simulink model "ss_inter_v3_i"  (R2019a)
settings: Solver=ode14x  StartTime=beginTime  StopTime=.3917  FixedStep=1e-4  RelTol=1e-3  EnableMultiTasking=on
model workspace (MAT data in the model file):
  Ankle_L_D = 1.86999822456
  Ankle_L_S = 0.0237763920936
  Ankle_R_D = 0.0588397140494
  Ankle_R_S = 0.739584271752
  F_C = 0.0618
  F_H = 0.107
  F_I = 0.0129
  F_L = 0.2471
  F_M = 1.2499
  F_W = 0.11
  GRF_HD = 42097.5090581
  GRF_HS = 111995.804745
  GRF_VD = 23523.4518935
  GRF_VS = 88551.3661398
  HAT_I = 4.3688
  HAT_L = 0.549
  HAT_M = 58.9182
  HAT_a = 0.2
  HAT_b = 0.13
  Hip_L_D = 0.00120944164738
  Hip_L_S = 1.91959156409
  Hip_R_D = 0.00174333284727
  Hip_R_S = 0.483982271561
  Knee_L_D = 0.900041230997
  Knee_L_S = 0.0187606009115
  Knee_R_D = 0.0722123401531
  Knee_R_S = 0.341684886913
  M : struct (value not decoded)
  S_I = 0.073
  S_L = 0.447
  S_M = 4.0083
  S_R1 = 0.06
  S_R2 = 0.08
  T_I = 0.2042
  T_L = 0.476
  T_M = 8.62
  T_R1 = 0.08
  T_R2 = 0.1
  beginTime = 0
  bodymass = 86.2
  lagStanceAnkle = [-99.7972 119.6384 39.1959 13.6502 4.806 38.9221]
  lagSwingAnkle = [13.6022 -2.7997 -4.4346 -3.8168 -10.7505 -9.0476]
  lagSwingHip = [-0.8171 -4.531 -6.5727 -10.5819 -21.4348 -39.6754]
  lagSwingKnee = [12.9765 10.8307 12.1552 13.6508 15.8758 16.223]
  p_stance_ankle_i = 1.9958
  p_stance_hip_i = -0.3323
  p_stance_knee_i = -0.8489
  p_swing_ankle_i = -0.4822
  p_swing_hip_i = -0.4475
  p_swing_knee_i = -0.4822
  polyfit_stance_ankle = [14817.0133912 -12307.4669363 2660.6079459 -392.465308084 -22.4679780976]
  polyfit_swing_ankle = [1827062.95885 -2490254.69612 1362128.66207 -378716.545114 54333.2821512 -3279.80936759 -14.4988961426 7.65411149052]
  polyfit_swing_hip = [-165694475.688 242689298.766 -143233708.247 44214448.7429 -7786254.41967 786446.146696 -39221.5649329 184.642317874 42.6030082642]
  polyfit_swing_knee = [-833880.523134 699128.406901 -179568.608041 9158.11345477 2208.69768841 -148.905653355 -15.7767198565]
  w_stance_ankle_i = 1.3
  w_stance_hip_i = 1.44372264721e-05
  w_stance_knee_i = 1.72097647422e-05
  w_swing_ankle_i = -2.2
  w_swing_hip_i = -0.00239916102262
  w_swing_knee_i = -0.00263690015709
  x_planar_p_i = 0
  x_planar_v_i = 0
  y_planar_p_i = 0
  y_planar_v_i = 0
  z_planar_p_i = 0
  z_planar_v_i = 0
values from neighbouring files (symbols this model uses):
  N = 3    [lagdmodel.m]
symbols that are objects in the model workspace (value not decoded): M
undefined symbols (not defined in the file or in its folder): X, Y, Z
libraries: nesl_utility x104, sm_lib x67, fl_lib x24, fl_ps_legacy_lib x14
(part 4 of 4)

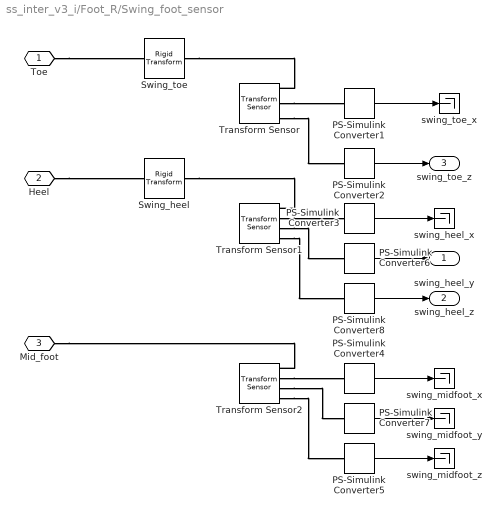
== system ss_inter_v3_i/Foot_R/Swing_foot_sensor ==
  PS-Simulink Converter{1..8} (8 alike) : nesl_utility/PS-Simulink Converter  PhysicalDomain=network_engine_domain  SubClassName=ps_output  LeftPortType=input  RightPortType=output  PseudoPeriodic=off  Frequencies=[]  Unit=1  AffineConversion=off
  Swing_heel : sm_lib/Frames and Transforms/Rigid Transform  TranslationMethod=StandardAxis  TranslationStandardOffset=F_C  TranslationLengthUnit=m  TranslationStandardAxis=-X  TranslationCartesianOffset=[0 0 0]  TranslationROffset=0  TranslationROffsetUnits=m  TranslationZOffset=0  TranslationZOffsetUnits=m  TranslationThetaOffset=0  TranslationThetaOffsetUnits=deg  RotationMethod=None  RotationAngleUnits=deg  RotationStandardAxis=+Z  RotationAngle=0  RotationArbitraryAxis=[0 0 1]  FollAlignAxisA=+X  BaseAlignAxisA=+Y  FollAlignAxisB=+Y  BaseAlignAxisB=+Z  RotationSequenceAxes=FollowerAxes  RotationSequence=XYX  RotationSequenceAngles=[0 0 0]  RotationSequenceAnglesUnits=deg  RotationMatrix=[1 0 0; 0 1 0; 0 0 1]
  Swing_toe : sm_lib/Frames and Transforms/Rigid Transform  TranslationMethod=StandardAxis  TranslationStandardOffset=F_L-F_C  TranslationLengthUnit=m  TranslationStandardAxis=+X  TranslationCartesianOffset=[0 0 0]  TranslationROffset=0  TranslationROffsetUnits=m  TranslationZOffset=0  TranslationZOffsetUnits=m  TranslationThetaOffset=0  TranslationThetaOffsetUnits=deg  RotationMethod=None  RotationAngleUnits=deg  RotationStandardAxis=+Z  RotationAngle=0  RotationArbitraryAxis=[0 0 1]  FollAlignAxisA=+X  BaseAlignAxisA=+Y  FollAlignAxisB=+Y  BaseAlignAxisB=+Z  RotationSequenceAxes=FollowerAxes  RotationSequence=XYX  RotationSequenceAngles=[0 0 0]  RotationSequenceAnglesUnits=deg  RotationMatrix=[1 0 0; 0 1 0; 0 0 1]
  Transform Sensor : sm_lib/Frames and Transforms/Transform Sensor  MeasurementFrame=World  SenseAngle=off  SenseAxis=off  SenseAngle1=off  SenseAngle2=off  SenseAngle3=off  SenseQ=off  SenseR=off  SenseOmegaX=off  SenseOmegaY=off  SenseOmegaZ=off  SenseOmega1=off  SenseOmega2=off  SenseOmega3=off  SenseQDot=off  SenseRDot=off  SenseAlphaX=off  SenseAlphaY=off  SenseAlphaZ=off  SenseAlpha1=off  SenseAlpha2=off  SenseAlpha3=off  SenseQDDot=off  SenseRDDot=off  SenseX=on  SenseY=off  SenseZ=on  SenseRad=off  SenseAzim=off  SenseDist=off  SenseInc=off  SenseXDot=off  SenseYDot=off  SenseZDot=off  SenseRadDot=off  SenseAzimDot=off  SenseDistDot=off  SenseIncDot=off  SenseXDDot=off  SenseYDDot=off  SenseZDDot=off  SenseRadDDot=off  SenseAzimDDot=off  SenseDistDDot=off  SenseIncDDot=off
  Transform Sensor1 : sm_lib/Frames and Transforms/Transform Sensor  MeasurementFrame=World  SenseAngle=off  SenseAxis=off  SenseAngle1=off  SenseAngle2=off  SenseAngle3=off  SenseQ=off  SenseR=off  SenseOmegaX=off  SenseOmegaY=off  SenseOmegaZ=off  SenseOmega1=off  SenseOmega2=off  SenseOmega3=off  SenseQDot=off  SenseRDot=off  SenseAlphaX=off  SenseAlphaY=off  SenseAlphaZ=off  SenseAlpha1=off  SenseAlpha2=off  SenseAlpha3=off  SenseQDDot=off  SenseRDDot=off  SenseX=on  SenseY=on  SenseZ=on  SenseRad=off  SenseAzim=off  SenseDist=off  SenseInc=off  SenseXDot=off  SenseYDot=off  SenseZDot=off  SenseRadDot=off  SenseAzimDot=off  SenseDistDot=off  SenseIncDot=off  SenseXDDot=off  SenseYDDot=off  SenseZDDot=off  SenseRadDDot=off  SenseAzimDDot=off  SenseDistDDot=off  SenseIncDDot=off
  Transform Sensor2 : sm_lib/Frames and Transforms/Transform Sensor  MeasurementFrame=World  SenseAngle=off  SenseAxis=off  SenseAngle1=off  SenseAngle2=off  SenseAngle3=off  SenseQ=off  SenseR=off  SenseOmegaX=off  SenseOmegaY=off  SenseOmegaZ=off  SenseOmega1=off  SenseOmega2=off  SenseOmega3=off  SenseQDot=off  SenseRDot=off  SenseAlphaX=off  SenseAlphaY=off  SenseAlphaZ=off  SenseAlpha1=off  SenseAlpha2=off  SenseAlpha3=off  SenseQDDot=off  SenseRDDot=off  SenseX=on  SenseY=on  SenseZ=on  SenseRad=off  SenseAzim=off  SenseDist=off  SenseInc=off  SenseXDot=off  SenseYDot=off  SenseZDot=off  SenseRadDot=off  SenseAzimDot=off  SenseDistDot=off  SenseIncDot=off  SenseXDDot=off  SenseYDDot=off  SenseZDDot=off  SenseRadDDot=off  SenseAzimDDot=off  SenseDistDDot=off  SenseIncDDot=off
  swing_heel_x : Terminator
  swing_midfoot_x : Terminator
  swing_midfoot_y : Terminator
  swing_midfoot_z : Terminator
  swing_toe_x : Terminator
  Toe : PMIOPort  Side=Left
  Heel : PMIOPort  Port=2  Side=Left
  Mid_foot : PMIOPort  Port=3  Side=Left
  swing_heel_y : Outport
  swing_heel_z : Outport  Port=2
  swing_toe_z : Outport  Port=3
  wires:
  PS-Simulink Converter1/1 -> swing_toe_x/1
  PS-Simulink Converter2/1 -> swing_toe_z/1
  PS-Simulink Converter3/1 -> swing_heel_x/1
  PS-Simulink Converter6/1 -> swing_heel_y/1
  PS-Simulink Converter4/1 -> swing_midfoot_x/1
  PS-Simulink Converter7/1 -> swing_midfoot_y/1
  PS-Simulink Converter5/1 -> swing_midfoot_z/1
  PS-Simulink Converter8/1 -> swing_heel_z/1
  connections:
  Swing_heel/RConn1 -- Transform Sensor1/RConn1
  Swing_toe/RConn1 -- Transform Sensor/RConn1
  Heel/RConn1 -- Swing_heel/LConn1
  Toe/RConn1 -- Swing_toe/LConn1
  Mid_foot/RConn1 -- Transform Sensor2/RConn1
  Transform Sensor2/RConn2 -- PS-Simulink Converter4/LConn1
  Transform Sensor/RConn2 -- PS-Simulink Converter1/LConn1
  Transform Sensor/RConn3 -- PS-Simulink Converter2/LConn1
  Transform Sensor1/RConn2 -- PS-Simulink Converter3/LConn1
  Transform Sensor1/RConn3 -- PS-Simulink Converter6/LConn1
  Transform Sensor2/RConn4 -- PS-Simulink Converter5/LConn1
  Transform Sensor2/RConn3 -- PS-Simulink Converter7/LConn1
  Transform Sensor1/RConn4 -- PS-Simulink Converter8/LConn1

== system ss_inter_v3_i/HAT/COMCal ==
  COM Energy Calc : Subsystem
  PS-S : nesl_utility/PS-Simulink Converter  PhysicalDomain=network_engine_domain  SubClassName=ps_output  LeftPortType=input  RightPortType=output  PseudoPeriodic=off  Frequencies=[]  Unit=1  AffineConversion=off
  Transform Sensor : sm_lib/Frames and Transforms/Transform Sensor  MeasurementFrame=World  SenseAngle=off  SenseAxis=off  SenseAngle1=off  SenseAngle2=off  SenseAngle3=off  SenseQ=off  SenseR=off  SenseOmegaX=off  SenseOmegaY=off  SenseOmegaZ=off  SenseOmega1=off  SenseOmega2=off  SenseOmega3=off  SenseQDot=off  SenseRDot=off  SenseAlphaX=off  SenseAlphaY=off  SenseAlphaZ=off  SenseAlpha1=off  SenseAlpha2=off  SenseAlpha3=off  SenseQDDot=off  SenseRDDot=off  SenseX=off  SenseY=off  SenseZ=on  SenseRad=off  SenseAzim=off  SenseDist=off  SenseInc=off  SenseXDot=on  SenseYDot=on  SenseZDot=on  SenseRadDot=off  SenseAzimDot=off  SenseDistDot=off  SenseIncDot=off  SenseXDDot=off  SenseYDDot=off  SenseZDDot=off  SenseRadDDot=off  SenseAzimDDot=off  SenseDistDDot=off  SenseIncDDot=off
  Conn2 : PMIOPort  Side=Left
  vCOM : Outport
  COM Energy : Outport  Port=2
  wires:
  COM Energy Calc/1(Out1) -> COM Energy/1
  PS-S/1 -> vCOM/1
  connections:
  COM Energy Calc/LConn4 -- Transform Sensor/RConn5
  COM Energy Calc/LConn2 -- Transform Sensor/RConn3
  COM Energy Calc/LConn1 -- Transform Sensor/RConn2
  Transform Sensor/RConn4 -- COM Energy Calc/LConn3 -- PS-S/LConn1
  Transform Sensor/RConn1 -- Conn2/RConn1

== system ss_inter_v3_i/Hip_L_Actuation/Hard_Stop_Hip_L ==
  Mechanical Rotational Reference : fl_lib/Mechanical/Rotational Elements/Mechanical Rotational Reference
  Rotational Simscape Intf (Library Block) : Subsystem
  Rotational Hard Stop : fl_lib/Mechanical/Rotational Elements/Rotational Hard Stop  upper_bnd=upper_bound rad  lower_bnd=lower_bound rad  stiff_up=contact_stiffness N*m/rad  stiff_low=contact_stiffness N*m/rad  D_up=contact_damping N*m/(rad/s)  D_low=contact_damping N*m/(rad/s)  model=3  transition=0.001 rad  w_specify=off  w_priority=None  w=0 rad/s  w_nominal_specify=off  w_nominal_unit=rad/s  w_nominal_value=1  t_specify=off  t_priority=None  t=0 N*m  t_nominal_specify=off  t_nominal_unit=N*m  t_nominal_value=1  phi_specify=on  phi_priority=High  phi=initial_angular_position rad  phi_nominal_specify=off  phi_nominal_unit=rad  phi_nominal_value=1
      settings: SourceProductName=Simscape  SourceProductBaseCode=SS
  T : PMIOPort  Side=Right
  w : PMIOPort  Port=2  Side=Left
  connections:
  Rotational Simscape Intf (Library Block)/LConn2 -- Rotational Hard Stop/LConn1 -- Mechanical Rotational Reference/LConn1
  Rotational Hard Stop/RConn1 -- Rotational Simscape Intf (Library Block)/RConn2
  w/RConn1 -- Rotational Simscape Intf (Library Block)/LConn1
  Rotational Simscape Intf (Library Block)/RConn1 -- T/RConn1

== system ss_inter_v3_i/Hip_R_Actuation/Hard_Stop_Hip_R ==
  Mechanical Rotational Reference : fl_lib/Mechanical/Rotational Elements/Mechanical Rotational Reference
  Rotational Simscape Intf (Library Block) : Subsystem
  Rotational Hard Stop : fl_lib/Mechanical/Rotational Elements/Rotational Hard Stop  upper_bnd=upper_bound rad  lower_bnd=lower_bound rad  stiff_up=contact_stiffness N*m/rad  stiff_low=contact_stiffness N*m/rad  D_up=contact_damping N*m/(rad/s)  D_low=contact_damping N*m/(rad/s)  model=3  transition=0.001 rad  w_specify=off  w_priority=None  w=0 rad/s  w_nominal_specify=off  w_nominal_unit=rad/s  w_nominal_value=1  t_specify=off  t_priority=None  t=0 N*m  t_nominal_specify=off  t_nominal_unit=N*m  t_nominal_value=1  phi_specify=on  phi_priority=High  phi=initial_angular_position rad  phi_nominal_specify=off  phi_nominal_unit=rad  phi_nominal_value=1
      settings: SourceProductName=Simscape  SourceProductBaseCode=SS
  T : PMIOPort  Side=Right
  w : PMIOPort  Port=2  Side=Left
  connections:
  Rotational Simscape Intf (Library Block)/LConn2 -- Rotational Hard Stop/LConn1 -- Mechanical Rotational Reference/LConn1
  Rotational Hard Stop/RConn1 -- Rotational Simscape Intf (Library Block)/RConn2
  w/RConn1 -- Rotational Simscape Intf (Library Block)/LConn1
  Rotational Simscape Intf (Library Block)/RConn1 -- T/RConn1

== system ss_inter_v3_i/Knee_L_Actuation/Hard_Stop_Knee_L ==
  Mechanical Rotational Reference : fl_lib/Mechanical/Rotational Elements/Mechanical Rotational Reference
  Rotational Simscape Intf (Library Block) : Subsystem
  Rotational Hard Stop : fl_lib/Mechanical/Rotational Elements/Rotational Hard Stop  upper_bnd=upper_bound rad  lower_bnd=lower_bound rad  stiff_up=contact_stiffness N*m/rad  stiff_low=contact_stiffness N*m/rad  D_up=contact_damping N*m/(rad/s)  D_low=contact_damping N*m/(rad/s)  model=3  transition=0.001 rad  w_specify=off  w_priority=None  w=0 rad/s  w_nominal_specify=off  w_nominal_unit=rad/s  w_nominal_value=1  t_specify=off  t_priority=None  t=0 N*m  t_nominal_specify=off  t_nominal_unit=N*m  t_nominal_value=1  phi_specify=on  phi_priority=High  phi=initial_angular_position rad  phi_nominal_specify=off  phi_nominal_unit=rad  phi_nominal_value=1
      settings: SourceProductName=Simscape  SourceProductBaseCode=SS
  T : PMIOPort  Side=Right
  w : PMIOPort  Port=2  Side=Left
  connections:
  Rotational Simscape Intf (Library Block)/RConn1 -- T/RConn1
  w/RConn1 -- Rotational Simscape Intf (Library Block)/LConn1
  Rotational Hard Stop/RConn1 -- Rotational Simscape Intf (Library Block)/RConn2
  Mechanical Rotational Reference/LConn1 -- Rotational Hard Stop/LConn1 -- Rotational Simscape Intf (Library Block)/LConn2

== system ss_inter_v3_i/Knee_R_Actuation/Hard_Stop_Knee_L1 ==
  Mechanical Rotational Reference : fl_lib/Mechanical/Rotational Elements/Mechanical Rotational Reference
  Rotational Simscape Intf (Library Block) : Subsystem
  Rotational Hard Stop : fl_lib/Mechanical/Rotational Elements/Rotational Hard Stop  upper_bnd=upper_bound rad  lower_bnd=lower_bound rad  stiff_up=contact_stiffness N*m/rad  stiff_low=contact_stiffness N*m/rad  D_up=contact_damping N*m/(rad/s)  D_low=contact_damping N*m/(rad/s)  model=3  transition=0.001 rad  w_specify=off  w_priority=None  w=0 rad/s  w_nominal_specify=off  w_nominal_unit=rad/s  w_nominal_value=1  t_specify=off  t_priority=None  t=0 N*m  t_nominal_specify=off  t_nominal_unit=N*m  t_nominal_value=1  phi_specify=on  phi_priority=High  phi=initial_angular_position rad  phi_nominal_specify=off  phi_nominal_unit=rad  phi_nominal_value=1
      settings: SourceProductName=Simscape  SourceProductBaseCode=SS
  T : PMIOPort  Side=Right
  w : PMIOPort  Port=2  Side=Left
  connections:
  Rotational Simscape Intf (Library Block)/RConn1 -- T/RConn1
  w/RConn1 -- Rotational Simscape Intf (Library Block)/LConn1
  Rotational Hard Stop/RConn1 -- Rotational Simscape Intf (Library Block)/RConn2
  Mechanical Rotational Reference/LConn1 -- Rotational Hard Stop/LConn1 -- Rotational Simscape Intf (Library Block)/LConn2

== system ss_inter_v3_i/Shank_L/COM Energy Calc1 ==
  Add : Sum  Inputs=3
  Add1 : Sum  Inputs=2
  Constant : Constant  Value=0.5*(S_M)
  Math Function : Math  Operator=square  SaturateOnIntegerOverflow=on
  Math Function1 : Math  Operator=square  SaturateOnIntegerOverflow=on
  Math Function2 : Math  Operator=square  SaturateOnIntegerOverflow=on
  PS-S{1..4} (4 alike) : nesl_utility/PS-Simulink Converter  PhysicalDomain=network_engine_domain  SubClassName=ps_output  LeftPortType=input  RightPortType=output  PseudoPeriodic=off  Frequencies=[]  Unit=1  AffineConversion=off
  Product : Product  Inputs=3
  Product1 : Product
  g : Constant  Value=9.81
  m : Constant  Value=S_M
  h : PMIOPort  Side=Left
  wx : PMIOPort  Port=2  Side=Left
  vy : PMIOPort  Port=3  Side=Left
  vz : PMIOPort  Port=4  Side=Left
  Out1 : Outport
  wires:
  g/1 -> Product/1
  PS-S2/1 -> Math Function1/1
  PS-S3/1 -> Math Function/1
  PS-S4/1 -> Math Function2/1
  Constant/1 -> Product1/2
  Math Function1/1 -> Add/3
  Add1/1 -> Out1/1
  Product1/1 -> Add1/2
  Math Function2/1 -> Add/1
  Add/1 -> Product1/1
  Math Function/1 -> Add/2
  m/1 -> Product/2
  PS-S1/1 -> Product/3
  Product/1 -> Add1/1
  connections:
  PS-S2/LConn1 -- vz/RConn1
  PS-S3/LConn1 -- vy/RConn1
  PS-S1/LConn1 -- h/RConn1
  PS-S4/LConn1 -- wx/RConn1

== system ss_inter_v3_i/Shank_R/COM Energy Calc1 ==
  Add : Sum  Inputs=3
  Add1 : Sum  Inputs=2
  Constant : Constant  Value=0.5*(S_M)
  Math Function : Math  Operator=square  SaturateOnIntegerOverflow=on
  Math Function1 : Math  Operator=square  SaturateOnIntegerOverflow=on
  Math Function2 : Math  Operator=square  SaturateOnIntegerOverflow=on
  PS-S{1..4} (4 alike) : nesl_utility/PS-Simulink Converter  PhysicalDomain=network_engine_domain  SubClassName=ps_output  LeftPortType=input  RightPortType=output  PseudoPeriodic=off  Frequencies=[]  Unit=1  AffineConversion=off
  Product : Product  Inputs=3
  Product1 : Product
  g : Constant  Value=9.81
  m : Constant  Value=S_M
  h : PMIOPort  Side=Left
  wx : PMIOPort  Port=2  Side=Left
  vy : PMIOPort  Port=3  Side=Left
  vz : PMIOPort  Port=4  Side=Left
  Out1 : Outport
  wires:
  g/1 -> Product/1
  PS-S2/1 -> Math Function1/1
  PS-S3/1 -> Math Function/1
  PS-S4/1 -> Math Function2/1
  Constant/1 -> Product1/2
  Math Function1/1 -> Add/3
  Add1/1 -> Out1/1
  Product1/1 -> Add1/2
  Math Function2/1 -> Add/1
  Add/1 -> Product1/1
  Math Function/1 -> Add/2
  m/1 -> Product/2
  PS-S1/1 -> Product/3
  Product/1 -> Add1/1
  connections:
  PS-S2/LConn1 -- vz/RConn1
  PS-S3/LConn1 -- vy/RConn1
  PS-S1/LConn1 -- h/RConn1
  PS-S4/LConn1 -- wx/RConn1

== system ss_inter_v3_i/Thigh_L/COM Energy Calc1 ==
  Add : Sum  Inputs=3
  Add1 : Sum  Inputs=2
  Constant : Constant  Value=0.5*(T_M)
  Math Function : Math  Operator=square  SaturateOnIntegerOverflow=on
  Math Function1 : Math  Operator=square  SaturateOnIntegerOverflow=on
  Math Function2 : Math  Operator=square  SaturateOnIntegerOverflow=on
  PS-S{1..4} (4 alike) : nesl_utility/PS-Simulink Converter  PhysicalDomain=network_engine_domain  SubClassName=ps_output  LeftPortType=input  RightPortType=output  PseudoPeriodic=off  Frequencies=[]  Unit=1  AffineConversion=off
  Product : Product  Inputs=3
  Product1 : Product
  g : Constant  Value=9.81
  m : Constant  Value=T_M
  h : PMIOPort  Side=Left
  wx : PMIOPort  Port=2  Side=Left
  vy : PMIOPort  Port=3  Side=Left
  vz : PMIOPort  Port=4  Side=Left
  Out1 : Outport
  wires:
  g/1 -> Product/1
  PS-S2/1 -> Math Function1/1
  PS-S3/1 -> Math Function/1
  PS-S4/1 -> Math Function2/1
  Constant/1 -> Product1/2
  Math Function1/1 -> Add/3
  Add1/1 -> Out1/1
  Product1/1 -> Add1/2
  Math Function2/1 -> Add/1
  Add/1 -> Product1/1
  Math Function/1 -> Add/2
  m/1 -> Product/2
  PS-S1/1 -> Product/3
  Product/1 -> Add1/1
  connections:
  PS-S2/LConn1 -- vz/RConn1
  PS-S3/LConn1 -- vy/RConn1
  PS-S1/LConn1 -- h/RConn1
  PS-S4/LConn1 -- wx/RConn1

== system ss_inter_v3_i/Thigh_R/COM Energy Calc1 ==
  Add : Sum  Inputs=3
  Add1 : Sum  Inputs=2
  Constant : Constant  Value=0.5*(T_M)
  Math Function : Math  Operator=square  SaturateOnIntegerOverflow=on
  Math Function1 : Math  Operator=square  SaturateOnIntegerOverflow=on
  Math Function2 : Math  Operator=square  SaturateOnIntegerOverflow=on
  PS-S{1..4} (4 alike) : nesl_utility/PS-Simulink Converter  PhysicalDomain=network_engine_domain  SubClassName=ps_output  LeftPortType=input  RightPortType=output  PseudoPeriodic=off  Frequencies=[]  Unit=1  AffineConversion=off
  Product : Product  Inputs=3
  Product1 : Product
  g : Constant  Value=9.81
  m : Constant  Value=T_M
  h : PMIOPort  Side=Left
  wx : PMIOPort  Port=2  Side=Left
  vy : PMIOPort  Port=3  Side=Left
  vz : PMIOPort  Port=4  Side=Left
  Out1 : Outport
  wires:
  g/1 -> Product/1
  PS-S2/1 -> Math Function1/1
  PS-S3/1 -> Math Function/1
  PS-S4/1 -> Math Function2/1
  Constant/1 -> Product1/2
  Math Function1/1 -> Add/3
  Add1/1 -> Out1/1
  Product1/1 -> Add1/2
  Math Function2/1 -> Add/1
  Add/1 -> Product1/1
  Math Function/1 -> Add/2
  m/1 -> Product/2
  PS-S1/1 -> Product/3
  Product/1 -> Add1/1
  connections:
  PS-S2/LConn1 -- vz/RConn1
  PS-S3/LConn1 -- vy/RConn1
  PS-S1/LConn1 -- h/RConn1
  PS-S4/LConn1 -- wx/RConn1

== system ss_inter_v3_i/Ankle_L_Actuation/Hard_Stop_Ankle_L/Rotational Simscape Intf (Library Block) ==
  Ideal Angular Velocity Source : fl_lib/Mechanical/Mechanical Sources/Ideal Angular Velocity Source
  Ideal Torque Sensor : fl_lib/Mechanical/Mechanical Sensors/Ideal Torque Sensor
  w : PMIOPort  Side=Left
  T : PMIOPort  Port=2  Side=Right
  R : PMIOPort  Port=3  Side=Left
  C : PMIOPort  Port=4  Side=Right
  connections:
  w/RConn1 -- Ideal Angular Velocity Source/RConn1
  T/RConn1 -- Ideal Torque Sensor/RConn2
  Ideal Torque Sensor/LConn1 -- Ideal Angular Velocity Source/RConn2
  R/RConn1 -- Ideal Angular Velocity Source/LConn1
  Ideal Torque Sensor/RConn1 -- C/RConn1

== system ss_inter_v3_i/Ankle_R_Actuation/Hard_Stop_Ankle_L1/Rotational Simscape Intf (Library Block) ==
  Ideal Angular Velocity Source : fl_lib/Mechanical/Mechanical Sources/Ideal Angular Velocity Source
  Ideal Torque Sensor : fl_lib/Mechanical/Mechanical Sensors/Ideal Torque Sensor
  w : PMIOPort  Side=Left
  T : PMIOPort  Port=2  Side=Right
  R : PMIOPort  Port=3  Side=Left
  C : PMIOPort  Port=4  Side=Right
  connections:
  w/RConn1 -- Ideal Angular Velocity Source/RConn1
  T/RConn1 -- Ideal Torque Sensor/RConn2
  Ideal Torque Sensor/LConn1 -- Ideal Angular Velocity Source/RConn2
  R/RConn1 -- Ideal Angular Velocity Source/LConn1
  Ideal Torque Sensor/RConn1 -- C/RConn1

== system ss_inter_v3_i/Foot_L/Heel_GRF/Subsystem ==
  Constant : Constant  Value=0
  Constant1 : Constant  Value=0
  Damping : Switch
  Gain : Gain  Gain=-GRF_VS
  Gain1 : Gain  Gain=-GRF_VD
  PS-Simulink Converter : nesl_utility/PS-Simulink Converter  PhysicalDomain=network_engine_domain  SubClassName=ps_output  LeftPortType=input  RightPortType=output  PseudoPeriodic=off  Frequencies=[]  Unit=1  AffineConversion=off
  PS-Simulink Converter1 : nesl_utility/PS-Simulink Converter  PhysicalDomain=network_engine_domain  SubClassName=ps_output  LeftPortType=input  RightPortType=output  PseudoPeriodic=off  Frequencies=[]  Unit=1  AffineConversion=off
  Scope : Scope
  Scope1 : Scope
  Scope2 : Scope
  Simulink-PS Converter : nesl_utility/Simulink-PS Converter  PhysicalDomain=network_engine_domain  SubClassName=ps_input  LeftPortType=input  RightPortType=output  PseudoPeriodic=off  Frequencies=[]  NoiseDistribution=none  NoiseParameters=[]  Unit=1  AffineConversion=off  FilteringAndDerivatives=zero  SimscapeFilterOrder=1  InputFilterTimeConstant=.001  UdotUserProvided=[]
  Spring : Switch
  Sum : Sum  Inputs=|++
  Vertical Force : PMIOPort  Side=Right
  Vertical Position : PMIOPort  Port=2  Side=Left
  Vertical Velocity : PMIOPort  Port=3  Side=Left
  wires:
  Damping/1 -> Sum/2
  Spring/1 -> Sum/1
  PS-Simulink Converter1/1 -> Scope1/1, Gain1/1
  Gain1/1 -> Damping/3
  Constant1/1 -> Damping/1
  Constant/1 -> Spring/1
  Gain/1 -> Spring/3
  PS-Simulink Converter/1 -> Scope/1, Gain/1, Damping/2, Spring/2
  Sum/1 -> Scope2/1, Simulink-PS Converter/1
  connections:
  Vertical Position/RConn1 -- PS-Simulink Converter/LConn1
  Vertical Velocity/RConn1 -- PS-Simulink Converter1/LConn1
  Simulink-PS Converter/RConn1 -- Vertical Force/RConn1

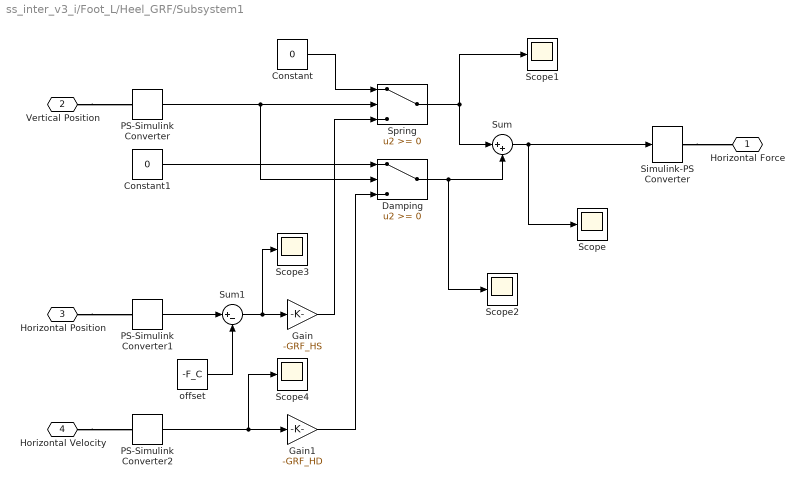
== system ss_inter_v3_i/Foot_L/Heel_GRF/Subsystem1 ==
  Constant : Constant  Value=0
  Constant1 : Constant  Value=0
  Damping : Switch
  Gain : Gain  Gain=-GRF_HS
  Gain1 : Gain  Gain=-GRF_HD
  PS-Simulink Converter : nesl_utility/PS-Simulink Converter  PhysicalDomain=network_engine_domain  SubClassName=ps_output  LeftPortType=input  RightPortType=output  PseudoPeriodic=off  Frequencies=[]  Unit=1  AffineConversion=off
  PS-Simulink Converter1 : nesl_utility/PS-Simulink Converter  PhysicalDomain=network_engine_domain  SubClassName=ps_output  LeftPortType=input  RightPortType=output  PseudoPeriodic=off  Frequencies=[]  Unit=1  AffineConversion=off
  PS-Simulink Converter2 : nesl_utility/PS-Simulink Converter  PhysicalDomain=network_engine_domain  SubClassName=ps_output  LeftPortType=input  RightPortType=output  PseudoPeriodic=off  Frequencies=[]  Unit=1  AffineConversion=off
  Scope{,1..4} (5 alike) : Scope
  Simulink-PS Converter : nesl_utility/Simulink-PS Converter  PhysicalDomain=network_engine_domain  SubClassName=ps_input  LeftPortType=input  RightPortType=output  PseudoPeriodic=off  Frequencies=[]  NoiseDistribution=none  NoiseParameters=[]  Unit=1  AffineConversion=off  FilteringAndDerivatives=zero  SimscapeFilterOrder=1  InputFilterTimeConstant=.001  UdotUserProvided=[]
  Spring : Switch
  Sum : Sum  Inputs=|++
  Sum1 : Sum  Inputs=|+-
  "offset " : Constant  Value=-F_C
  Horizontal Force : PMIOPort  Side=Right
  Vertical Position : PMIOPort  Port=2  Side=Left
  Horizontal Position : PMIOPort  Port=3  Side=Left
  Horizontal Velocity : PMIOPort  Port=4  Side=Left
  wires:
  PS-Simulink Converter/1 -> Spring/2, Damping/2
  Constant/1 -> Spring/1
  Spring/1 -> Scope1/1, Sum/1
  Damping/1 -> Scope2/1, Sum/2
  Constant1/1 -> Damping/1
  PS-Simulink Converter2/1 -> Scope4/1, Gain1/1
  Gain/1 -> Spring/3
  Gain1/1 -> Damping/3
  PS-Simulink Converter1/1 -> Sum1/1
  "offset "/1 -> Sum1/2
  Sum1/1 -> Scope3/1, Gain/1
  Sum/1 -> Simulink-PS Converter/1, Scope/1
  connections:
  Vertical Position/RConn1 -- PS-Simulink Converter/LConn1
  Horizontal Position/RConn1 -- PS-Simulink Converter1/LConn1
  Horizontal Velocity/RConn1 -- PS-Simulink Converter2/LConn1
  Simulink-PS Converter/RConn1 -- Horizontal Force/RConn1

== system ss_inter_v3_i/Foot_L/Toe_GRF/Subsystem ==
  Constant : Constant  Value=0
  Constant1 : Constant  Value=0
  Damping : Switch
  Gain : Gain  Gain=-GRF_VS
  Gain1 : Gain  Gain=-GRF_VD
  PS-Simulink Converter : nesl_utility/PS-Simulink Converter  PhysicalDomain=network_engine_domain  SubClassName=ps_output  LeftPortType=input  RightPortType=output  PseudoPeriodic=off  Frequencies=[]  Unit=1  AffineConversion=off
  PS-Simulink Converter1 : nesl_utility/PS-Simulink Converter  PhysicalDomain=network_engine_domain  SubClassName=ps_output  LeftPortType=input  RightPortType=output  PseudoPeriodic=off  Frequencies=[]  Unit=1  AffineConversion=off
  Scope : Scope
  Scope1 : Scope
  Scope2 : Scope
  Simulink-PS Converter : nesl_utility/Simulink-PS Converter  PhysicalDomain=network_engine_domain  SubClassName=ps_input  LeftPortType=input  RightPortType=output  PseudoPeriodic=off  Frequencies=[]  NoiseDistribution=none  NoiseParameters=[]  Unit=1  AffineConversion=off  FilteringAndDerivatives=zero  SimscapeFilterOrder=1  InputFilterTimeConstant=.001  UdotUserProvided=[]
  Spring : Switch
  Sum : Sum  Inputs=|++
  Vertical Force : PMIOPort  Side=Right
  Vertical Position : PMIOPort  Port=2  Side=Left
  Vertical Velocity : PMIOPort  Port=3  Side=Left
  wires:
  Damping/1 -> Sum/2
  Spring/1 -> Sum/1
  Sum/1 -> Scope2/1, Simulink-PS Converter/1
  PS-Simulink Converter1/1 -> Scope1/1, Gain1/1
  Gain1/1 -> Damping/3
  Constant1/1 -> Damping/1
  Constant/1 -> Spring/1
  Gain/1 -> Spring/3
  PS-Simulink Converter/1 -> Scope/1, Gain/1, Damping/2, Spring/2
  connections:
  Vertical Position/RConn1 -- PS-Simulink Converter/LConn1
  Vertical Velocity/RConn1 -- PS-Simulink Converter1/LConn1
  Simulink-PS Converter/RConn1 -- Vertical Force/RConn1

== system ss_inter_v3_i/Foot_L/Toe_GRF/Subsystem1 ==
  Constant : Constant  Value=0
  Constant1 : Constant  Value=0
  Damping : Switch
  Gain : Gain  Gain=-GRF_HS
  Gain1 : Gain  Gain=-GRF_HD
  PS-Simulink Converter : nesl_utility/PS-Simulink Converter  PhysicalDomain=network_engine_domain  SubClassName=ps_output  LeftPortType=input  RightPortType=output  PseudoPeriodic=off  Frequencies=[]  Unit=1  AffineConversion=off
  PS-Simulink Converter1 : nesl_utility/PS-Simulink Converter  PhysicalDomain=network_engine_domain  SubClassName=ps_output  LeftPortType=input  RightPortType=output  PseudoPeriodic=off  Frequencies=[]  Unit=1  AffineConversion=off
  PS-Simulink Converter2 : nesl_utility/PS-Simulink Converter  PhysicalDomain=network_engine_domain  SubClassName=ps_output  LeftPortType=input  RightPortType=output  PseudoPeriodic=off  Frequencies=[]  Unit=1  AffineConversion=off
  Scope : Scope
  Simulink-PS Converter : nesl_utility/Simulink-PS Converter  PhysicalDomain=network_engine_domain  SubClassName=ps_input  LeftPortType=input  RightPortType=output  PseudoPeriodic=off  Frequencies=[]  NoiseDistribution=none  NoiseParameters=[]  Unit=1  AffineConversion=off  FilteringAndDerivatives=zero  SimscapeFilterOrder=1  InputFilterTimeConstant=.001  UdotUserProvided=[]
  Spring : Switch
  Sum : Sum  Inputs=|++
  Sum1 : Sum  Inputs=|+-
  "offset " : Constant  Value=F_L-F_C
  Horizontal Force : PMIOPort  Side=Right
  Vertical Position : PMIOPort  Port=2  Side=Left
  Horizontal Position : PMIOPort  Port=3  Side=Left
  Horizontal Velocity : PMIOPort  Port=4  Side=Left
  wires:
  PS-Simulink Converter/1 -> Spring/2, Damping/2
  Constant/1 -> Spring/1
  Sum/1 -> Scope/1, Simulink-PS Converter/1
  Spring/1 -> Sum/1
  Damping/1 -> Sum/2
  Constant1/1 -> Damping/1
  PS-Simulink Converter2/1 -> Gain1/1
  Gain/1 -> Spring/3
  Gain1/1 -> Damping/3
  PS-Simulink Converter1/1 -> Sum1/1
  "offset "/1 -> Sum1/2
  Sum1/1 -> Gain/1
  connections:
  Vertical Position/RConn1 -- PS-Simulink Converter/LConn1
  Horizontal Position/RConn1 -- PS-Simulink Converter1/LConn1
  Horizontal Velocity/RConn1 -- PS-Simulink Converter2/LConn1
  Simulink-PS Converter/RConn1 -- Horizontal Force/RConn1

== system ss_inter_v3_i/HAT/COMCal/COM Energy Calc ==
  Add : Sum  Inputs=3
  Add1 : Sum  Inputs=2
  Constant : Constant  Value=0.5*(bodymass)
  Math Function : Math  Operator=square  SaturateOnIntegerOverflow=on
  Math Function1 : Math  Operator=square  SaturateOnIntegerOverflow=on
  Math Function2 : Math  Operator=square  SaturateOnIntegerOverflow=on
  PS-S{1..4} (4 alike) : nesl_utility/PS-Simulink Converter  PhysicalDomain=network_engine_domain  SubClassName=ps_output  LeftPortType=input  RightPortType=output  PseudoPeriodic=off  Frequencies=[]  Unit=1  AffineConversion=off
  Product : Product  Inputs=3
  Product1 : Product
  g : Constant  Value=9.81
  m : Constant  Value=bodymass
  h : PMIOPort  Side=Left
  vx : PMIOPort  Port=2  Side=Left
  vy : PMIOPort  Port=3  Side=Left
  vz : PMIOPort  Port=4  Side=Left
  Out1 : Outport
  wires:
  Product/1 -> Add1/1
  g/1 -> Product/1
  PS-S2/1 -> Math Function1/1
  PS-S3/1 -> Math Function/1
  PS-S4/1 -> Math Function2/1
  Constant/1 -> Product1/2
  Math Function1/1 -> Add/3
  Add1/1 -> Out1/1
  Product1/1 -> Add1/2
  Math Function2/1 -> Add/1
  Add/1 -> Product1/1
  Math Function/1 -> Add/2
  m/1 -> Product/2
  PS-S1/1 -> Product/3
  connections:
  PS-S2/LConn1 -- vz/RConn1
  PS-S3/LConn1 -- vy/RConn1
  PS-S1/LConn1 -- h/RConn1
  PS-S4/LConn1 -- vx/RConn1

== system ss_inter_v3_i/Hip_L_Actuation/Hard_Stop_Hip_L/Rotational Simscape Intf (Library Block) ==
  Ideal Angular Velocity Source : fl_lib/Mechanical/Mechanical Sources/Ideal Angular Velocity Source
  Ideal Torque Sensor : fl_lib/Mechanical/Mechanical Sensors/Ideal Torque Sensor
  w : PMIOPort  Side=Left
  T : PMIOPort  Port=2  Side=Right
  R : PMIOPort  Port=3  Side=Left
  C : PMIOPort  Port=4  Side=Right
  connections:
  w/RConn1 -- Ideal Angular Velocity Source/RConn1
  T/RConn1 -- Ideal Torque Sensor/RConn2
  Ideal Torque Sensor/LConn1 -- Ideal Angular Velocity Source/RConn2
  R/RConn1 -- Ideal Angular Velocity Source/LConn1
  Ideal Torque Sensor/RConn1 -- C/RConn1

== system ss_inter_v3_i/Hip_R_Actuation/Hard_Stop_Hip_R/Rotational Simscape Intf (Library Block) ==
  Ideal Angular Velocity Source : fl_lib/Mechanical/Mechanical Sources/Ideal Angular Velocity Source
  Ideal Torque Sensor : fl_lib/Mechanical/Mechanical Sensors/Ideal Torque Sensor
  w : PMIOPort  Side=Left
  T : PMIOPort  Port=2  Side=Right
  R : PMIOPort  Port=3  Side=Left
  C : PMIOPort  Port=4  Side=Right
  connections:
  w/RConn1 -- Ideal Angular Velocity Source/RConn1
  T/RConn1 -- Ideal Torque Sensor/RConn2
  Ideal Torque Sensor/LConn1 -- Ideal Angular Velocity Source/RConn2
  R/RConn1 -- Ideal Angular Velocity Source/LConn1
  Ideal Torque Sensor/RConn1 -- C/RConn1

== system ss_inter_v3_i/Knee_L_Actuation/Hard_Stop_Knee_L/Rotational Simscape Intf (Library Block) ==
  Ideal Angular Velocity Source : fl_lib/Mechanical/Mechanical Sources/Ideal Angular Velocity Source
  Ideal Torque Sensor : fl_lib/Mechanical/Mechanical Sensors/Ideal Torque Sensor
  w : PMIOPort  Side=Left
  T : PMIOPort  Port=2  Side=Right
  R : PMIOPort  Port=3  Side=Left
  C : PMIOPort  Port=4  Side=Right
  connections:
  Ideal Torque Sensor/RConn1 -- C/RConn1
  R/RConn1 -- Ideal Angular Velocity Source/LConn1
  Ideal Torque Sensor/LConn1 -- Ideal Angular Velocity Source/RConn2
  T/RConn1 -- Ideal Torque Sensor/RConn2
  w/RConn1 -- Ideal Angular Velocity Source/RConn1

== system ss_inter_v3_i/Knee_R_Actuation/Hard_Stop_Knee_L1/Rotational Simscape Intf (Library Block) ==
  Ideal Angular Velocity Source : fl_lib/Mechanical/Mechanical Sources/Ideal Angular Velocity Source
  Ideal Torque Sensor : fl_lib/Mechanical/Mechanical Sensors/Ideal Torque Sensor
  w : PMIOPort  Side=Left
  T : PMIOPort  Port=2  Side=Right
  R : PMIOPort  Port=3  Side=Left
  C : PMIOPort  Port=4  Side=Right
  connections:
  Ideal Torque Sensor/RConn1 -- C/RConn1
  R/RConn1 -- Ideal Angular Velocity Source/LConn1
  Ideal Torque Sensor/LConn1 -- Ideal Angular Velocity Source/RConn2
  T/RConn1 -- Ideal Torque Sensor/RConn2
  w/RConn1 -- Ideal Angular Velocity Source/RConn1
